simulink library "RobotG18_Blocos"  (R2016a)
settings: Solver=VariableStepAuto  StartTime=0.0  StopTime=10.0  RelTol=1e-3
settings Model: Creator=Catarina  LastModifiedBy=Catarina
settings GRTTargetCC: GeneratePreprocessorConditionals=Use local settings

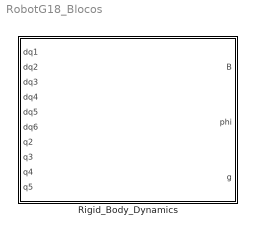
== system RobotG18_Blocos ==
  Rigid_Body_Dynamics : MATLAB Function  TreatAsAtomicUnit=on

== matlab function RobotG18_Blocos/Rigid_Body_Dynamics ==
  data: dq1 input; B output; dq2 input; dq3 input; dq4 input; dq5 input; dq6 input; q2 input; q3 input; q4 input; q5 input; phi output; g output
function [B,phi,g] = Rigid_Body_Dynamics(dq1,dq2,dq3,dq4,dq5,dq6,q2,q3,q4,q5)
%#codegen

%    This function was generated by the Symbolic Math Toolbox version 7.0.
%    17-May-2021 21:26:31

t2 = q2.*2.0;
t3 = q3.*2.0;
t4 = q4.*2.0;
t5 = q5.*2.0;
t6 = q2+q3+q4;
t7 = cos(t6);
t8 = q2+q3+q5;
t9 = sin(t8);
t10 = q2+q3-q5;
t11 = sin(t10);
t12 = q2+q3+q4+q5;
t13 = cos(t12);
t14 = t13.*2.24434e-4;
t15 = q2+q3;
t16 = sin(t15);
t17 = q2+q3+q4-q5;
t18 = cos(t17);
t19 = q2+q3+q4-t5;
t20 = cos(t19);
t21 = q2+q3+q4+t5;
t22 = cos(t21);
t23 = t22.*1.004271e-3;
t24 = q2-q5;
t25 = sin(t24);
t26 = q2+q5;
t27 = sin(t26);
t28 = t9.*6.284152e-3;
t29 = t27.*6.813175e-3;
t30 = sin(q2);
t31 = q4-q5;
t32 = sin(t31);
t33 = q3+q4+q5;
t34 = sin(t33);
t35 = cos(t5);
t36 = q3+q4-q5;
t37 = sin(t36);
t38 = q3+q4;
t39 = sin(t38);
t40 = q4+q5;
t41 = sin(t40);
t42 = cos(q3);
t43 = sin(q4);
t44 = t34.*6.813175e-3;
t45 = t41.*1.2568304e-2;
t46 = t42.*5.92297e-1;
t47 = t41.*6.284152e-3;
t48 = cos(q5);
t49 = t37.*6.813175e-3;
t50 = t32.*6.284152e-3;
t51 = t48.*2.75e-4;
t52 = t7.*(-8.11832e-3)+t14-t18.*3.270324e-3-t20.*1.004271e-3+t23;
t54 = t35.*2.008542e-3;
t53 = t43.*(-2.919616e-2)+t47-t50-t54+1.0090142e-2;
t55 = t7.*4.561084e-3;
t56 = t13.*3.270324e-3;
t57 = t18.*2.24434e-4;
t58 = t11.*(-6.284152e-3)-t25.*6.813175e-3+t28+t29+t55+t56+t57;
t60 = t48.*3.04589e-3;
t59 = t44+t47+t49+t50-t60;
t61 = dq2.^2;
t62 = sin(t17);
t63 = dq3.^2;
t64 = sin(t19);
t65 = sin(t21);
t66 = dq4.^2;
t67 = dq5.^2;
t68 = cos(t24);
t69 = cos(t8);
t70 = sin(t6);
t71 = cos(t10);
t72 = sin(t12);
t73 = cos(t15);
t74 = cos(t26);
t75 = sin(q5);
t76 = q3+q4+q5+t2;
t77 = cos(t76);
t78 = cos(t31);
t79 = q3+t2;
t80 = sin(t79);
t81 = -q5+t2+t3+t4;
t82 = t2+t3+t4+t5;
t83 = sin(t81);
t84 = t2+t3+t4-t5;
t85 = sin(t84);
t86 = sin(t82);
t87 = cos(t33);
t88 = t2+t3+t4;
t89 = sin(t88);
t90 = q3+q4-q5+t2;
t91 = q4+q5+t2+t3;
t92 = cos(t90);
t93 = cos(t91);
t94 = t2+t3;
t95 = sin(t94);
t96 = q3+q4+t2;
t97 = cos(t96);
t98 = cos(t36);
t99 = cos(t38);
t100 = cos(t40);
t101 = q4-q5+t2+t3;
t102 = cos(t101);
t103 = q5+t2+t3+t4;
t104 = sin(t103);
t105 = q4+t2+t3;
B = reshape([t32.*(-6.284152e-3)+t35.*1.004271e-3-t37.*6.813175e-3-t39.*3.1654e-2-t43.*2.919616e-2+t44+t46+t47+t48.*6.989516e-3+cos(t2).*1.2343024296875+cos(t79).*5.92297e-1-cos(t81).*1.522945e-3-cos(t82).*5.021355e-4-cos(t88).*2.630029e-3+cos(t94).*4.3975568975e-1+cos(t103).*1.522945e-3+sin(t76).*6.813175e-3-sin(t90).*6.813175e-3+sin(t91).*6.284152e-3-sin(t96).*3.1654e-2-sin(t101).*6.284152e-3-sin(t105).*2.919616e-2-cos(q5.*-2.0+t2+t3+t4).*5.021355e-4+1.8244887907375,t7.*(-8.11832e-3)-t11.*6.284152e-3+t14-t16.*6.2876312e-2-t18.*3.270324e-3-t20.*1.004271e-3+t23-t25.*6.813175e-3-t28-t29-t30.*2.9199618625e-1,t7.*(-8.11832e-3)-t11.*6.284152e-3+t14-t16.*6.2876312e-2-t18.*3.270324e-3-t20.*1.004271e-3+t23-t28,t52,t58,t70.*t75.*2.75e-4,t7.*(-8.11832e-3)-t9.*6.284152e-3-t11.*6.284152e-3+t14-t16.*6.2876312e-2-t18.*3.270324e-3-t20.*1.004271e-3+t23-t25.*6.813175e-3-t27.*6.813175e-3-t30.*2.9199618625e-1,t32.*(-1.2568304e-2)+t34.*1.362635e-2-t35.*2.008542e-3-t37.*1.362635e-2-t39.*6.3308e-2+t42.*1.184594-t43.*5.839232e-2+t45+3.377115380875,t32.*(-1.2568304e-2)-t35.*2.008542e-3-t39.*3.1654e-2-t43.*5.839232e-2+t44+t45+t46-t49+8.953005215e-1,t35.*(-2.008542e-3)-t39.*3.1654e-2-t43.*2.919616e-2+t44+t47-t49-t50+1.0090142e-2,t59,t51,t7.*(-8.11832e-3)-t9.*6.284152e-3-t11.*6.284152e-3+t14-t16.*6.2876312e-2-t18.*3.270324e-3-t20.*1.004271e-3+t23,t32.*(-1.2568304e-2)-t35.*2.008542e-3-t37.*6.813175e-3-t39.*3.1654e-2-t43.*5.839232e-2+t44+t45+t46+8.953005215e-1,t32.*(-1.2568304e-2)-t35.*2.008542e-3-t43.*5.839232e-2+t45+8.953005215e-1,t53,t47+t50-t60,t51,t52,t32.*(-6.284152e-3)-t35.*2.008542e-3-t37.*6.813175e-3-t39.*3.1654e-2-t43.*2.919616e-2+t44+t47+1.0090142e-2,t53,-t54+1.0090142e-2,-t60,t51,t58,t59,t47-t48.*3.04589e-3+t50,t48.*(-3.04589e-3),4.561084e-3,0.0,t13.*(-1.375e-4)+t18.*1.375e-4,t51,t51,t51,0.0,2.75e-4],[6,6]);
if nargout > 1
    t106 = cos(t105);
    t107 = sin(q3);
    t108 = dq1.^2;
    t109 = sin(t2);
    t110 = cos(q4);
    t111 = sin(t5);
    t112 = t67.*t75.*3.04589e-3;
    t113 = t95.*t108.*4.3975568975e-1;
    t114 = t66.*t100.*6.284152e-3;
    t115 = t67.*t100.*6.284152e-3;
    t116 = t102.*t108.*6.284152e-3;
    t117 = t104.*t108.*1.522945e-3;
    t118 = t106.*t108.*2.919616e-2;
    t119 = dq1.*dq6.*t62.*1.375e-4;
    t120 = dq2.*dq5.*t78.*1.2568304e-2;
    t121 = dq3.*dq5.*t78.*1.2568304e-2;
    t122 = dq4.*dq5.*t78.*1.2568304e-2;
    t123 = dq1.*dq5.*t70.*4.561084e-3;
    t124 = dq2.*dq5.*t111.*4.017084e-3;
    t125 = dq3.*dq5.*t111.*4.017084e-3;
    t126 = dq4.*dq5.*t111.*4.017084e-3;
    t127 = dq1.*dq5.*t71.*1.2568304e-2;
    t128 = dq1.*dq5.*t72.*3.04589e-3;
    t129 = dq2.*dq4.*t100.*1.2568304e-2;
    t130 = dq2.*dq5.*t100.*1.2568304e-2;
    t131 = dq3.*dq4.*t100.*1.2568304e-2;
    t132 = dq3.*dq5.*t100.*1.2568304e-2;
    t133 = dq4.*dq5.*t100.*1.2568304e-2;
    t134 = t92.*t108.*3.4065875e-3;
    t135 = t97.*t108.*1.5827e-2;
    t136 = t98.*t108.*3.4065875e-3;
    t137 = t61.*t98.*6.813175e-3;
    t138 = t99.*t108.*1.5827e-2;
    t139 = t61.*t99.*3.1654e-2;
    t140 = t78.*t108.*3.142076e-3;
    t141 = t61.*t78.*6.284152e-3;
    t142 = t63.*t78.*6.284152e-3;
    t143 = t102.*t108.*3.142076e-3;
    t144 = dq2.*dq3.*t78.*1.2568304e-2;
    t145 = cos(q2);
    phi = [t61.*t62.*3.270324e-3+t61.*t64.*1.004271e-3+t62.*t63.*3.270324e-3-t61.*t65.*1.004271e-3+t63.*t64.*1.004271e-3+t62.*t66.*3.270324e-3-t63.*t65.*1.004271e-3-t61.*t68.*6.813175e-3+t62.*t67.*2.24434e-4-t61.*t69.*6.284152e-3+t64.*t66.*1.004271e-3+t61.*t70.*8.11832e-3-t65.*t66.*1.004271e-3-t61.*t71.*6.284152e-3-t63.*t69.*6.284152e-3-t61.*t72.*2.24434e-4+t63.*t70.*8.11832e-3-t61.*t73.*6.2876312e-2-t63.*t71.*6.284152e-3-t61.*t74.*6.813175e-3-t63.*t72.*2.24434e-4+t67.*t68.*6.813175e-3-t63.*t73.*6.2876312e-2+t66.*t70.*8.11832e-3+t67.*t69.*6.284152e-3-t66.*t72.*2.24434e-4+t67.*t71.*6.284152e-3-t67.*t72.*3.270324e-3+t67.*t74.*6.813175e-3-t61.*t145.*2.9199618625e-1+dq2.*dq3.*t62.*6.540648e-3+dq2.*dq4.*t62.*6.540648e-3+dq2.*dq3.*t64.*2.008542e-3-dq2.*dq5.*t62.*3.494758e-3+dq3.*dq4.*t62.*6.540648e-3-dq2.*dq3.*t65.*2.008542e-3+dq2.*dq4.*t64.*2.008542e-3-dq2.*dq6.*t62.*1.375e-4-dq3.*dq5.*t62.*3.494758e-3-dq2.*dq4.*t65.*2.008542e-3-dq2.*dq5.*t64.*2.008542e-3+dq3.*dq4.*t64.*2.008542e-3-dq3.*dq6.*t62.*1.375e-4-dq4.*dq5.*t62.*3.494758e-3-dq2.*dq5.*t65.*2.008542e-3-dq3.*dq4.*t65.*2.008542e-3-dq3.*dq5.*t64.*2.008542e-3-dq4.*dq6.*t62.*1.375e-4-dq3.*dq5.*t65.*2.008542e-3-dq4.*dq5.*t64.*2.008542e-3+dq5.*dq6.*t62.*1.375e-4-dq2.*dq3.*t69.*1.2568304e-2-dq4.*dq5.*t65.*2.008542e-3+dq2.*dq3.*t70.*1.623664e-2-dq2.*dq3.*t71.*1.2568304e-2+dq2.*dq4.*t70.*1.623664e-2-dq2.*dq3.*t72.*4.48868e-4-dq2.*dq5.*t70.*4.561084e-3+dq3.*dq4.*t70.*1.623664e-2-dq2.*dq3.*t73.*1.25752624e-1-dq2.*dq4.*t72.*4.48868e-4-dq3.*dq5.*t70.*4.561084e-3-dq2.*dq5.*t72.*3.494758e-3-dq3.*dq4.*t72.*4.48868e-4-dq4.*dq5.*t70.*4.561084e-3+dq1.*dq2.*t77.*1.362635e-2+dq2.*dq6.*t72.*1.375e-4-dq3.*dq5.*t72.*3.494758e-3+dq1.*dq3.*t77.*6.813175e-3-dq1.*dq5.*t75.*6.989516e-3+dq3.*dq6.*t72.*1.375e-4-dq4.*dq5.*t72.*3.494758e-3+dq1.*dq4.*t77.*6.813175e-3+dq4.*dq6.*t72.*1.375e-4-dq1.*dq2.*t80.*1.184594-dq1.*dq4.*t78.*6.284152e-3+dq1.*dq5.*t77.*6.813175e-3+dq5.*dq6.*t72.*1.375e-4-dq1.*dq3.*t80.*5.92297e-1+dq1.*dq5.*t78.*6.284152e-3+dq1.*dq2.*t83.*3.04589e-3+dq1.*dq3.*t83.*3.04589e-3+dq1.*dq2.*t85.*1.004271e-3+dq1.*dq4.*t83.*3.04589e-3+dq1.*dq2.*t86.*1.004271e-3+dq1.*dq3.*t85.*1.004271e-3-dq1.*dq5.*t83.*1.522945e-3+dq1.*dq3.*t86.*1.004271e-3+dq1.*dq4.*t85.*1.004271e-3+dq1.*dq3.*t87.*6.813175e-3+dq1.*dq4.*t86.*1.004271e-3-dq1.*dq5.*t85.*1.004271e-3+dq1.*dq2.*t89.*5.260058e-3+dq1.*dq4.*t87.*6.813175e-3+dq1.*dq5.*t86.*1.004271e-3+dq1.*dq3.*t89.*5.260058e-3+dq1.*dq5.*t87.*6.813175e-3+dq1.*dq4.*t89.*5.260058e-3-dq1.*dq2.*t92.*1.362635e-2+dq1.*dq2.*t93.*1.2568304e-2-dq1.*dq3.*t92.*6.813175e-3+dq1.*dq3.*t93.*1.2568304e-2-dq1.*dq4.*t92.*6.813175e-3-dq1.*dq2.*t95.*8.795113794999999e-1+dq1.*dq4.*t93.*6.284152e-3+dq1.*dq5.*t92.*6.813175e-3-dq1.*dq3.*t95.*8.795113794999999e-1+dq1.*dq5.*t93.*6.284152e-3-dq1.*dq2.*t97.*6.3308e-2-dq1.*dq3.*t97.*3.1654e-2-dq1.*dq3.*t98.*6.813175e-3-dq1.*dq4.*t97.*3.1654e-2-dq1.*dq3.*t99.*3.1654e-2-dq1.*dq4.*t98.*6.813175e-3-dq1.*dq4.*t99.*3.1654e-2+dq1.*dq5.*t98.*6.813175e-3-dq1.*dq2.*t102.*1.2568304e-2+dq1.*dq4.*t100.*6.284152e-3-dq1.*dq3.*t102.*1.2568304e-2+dq1.*dq5.*t100.*6.284152e-3-dq1.*dq2.*t104.*3.04589e-3-dq1.*dq4.*t102.*6.284152e-3-dq1.*dq3.*t104.*3.04589e-3+dq1.*dq5.*t102.*6.284152e-3-dq1.*dq2.*t106.*5.839232e-2-dq1.*dq4.*t104.*3.04589e-3-dq1.*dq3.*t106.*5.839232e-2-dq1.*dq5.*t104.*1.522945e-3-dq1.*dq3.*t107.*5.92297e-1-dq1.*dq4.*t106.*2.919616e-2-dq1.*dq2.*t109.*2.468604859375-dq1.*dq4.*t110.*2.919616e-2-dq1.*dq5.*t111.*2.008542e-3;t112+t113+t114+t115+t116+t117+t118+t119+t120+t121+t122+t123+t124+t125+t126+t127+t128+t129+t130+t131+t132+t133-t66.*t78.*6.284152e-3-t67.*t78.*6.284152e-3+t63.*t87.*6.813175e-3+t66.*t87.*6.813175e-3+t67.*t87.*6.813175e-3-t63.*t98.*6.813175e-3-t63.*t99.*3.1654e-2-t66.*t98.*6.813175e-3-t66.*t99.*3.1654e-2-t67.*t98.*6.813175e-3-t63.*t107.*5.92297e-1-t66.*t110.*2.919616e-2-t77.*t108.*6.813175e-3+t80.*t108.*5.92297e-1-t83.*t108.*1.522945e-3-t85.*t108.*5.021355e-4-t86.*t108.*5.021355e-4-t89.*t108.*2.630029e-3+t92.*t108.*6.813175e-3-t93.*t108.*6.284152e-3+t97.*t108.*3.1654e-2+t108.*t109.*1.2343024296875-dq1.*dq5.*t62.*3.04589e-3-dq1.*dq5.*t64.*2.008542e-3-dq1.*dq5.*t65.*2.008542e-3+dq1.*dq5.*t68.*1.362635e-2-dq1.*dq5.*t69.*1.2568304e-2-dq1.*dq6.*t72.*1.375e-4-dq1.*dq5.*t74.*1.362635e-2-dq2.*dq4.*t78.*1.2568304e-2-dq3.*dq4.*t78.*1.2568304e-2-dq5.*dq6.*t75.*2.75e-4+dq2.*dq3.*t87.*1.362635e-2+dq2.*dq4.*t87.*1.362635e-2+dq2.*dq5.*t87.*1.362635e-2+dq3.*dq4.*t87.*1.362635e-2+dq3.*dq5.*t87.*1.362635e-2+dq4.*dq5.*t87.*1.362635e-2-dq2.*dq3.*t98.*1.362635e-2-dq2.*dq3.*t99.*6.3308e-2-dq2.*dq4.*t98.*1.362635e-2-dq2.*dq4.*t99.*6.3308e-2+dq2.*dq5.*t98.*1.362635e-2-dq3.*dq4.*t98.*1.362635e-2-dq3.*dq4.*t99.*6.3308e-2+dq3.*dq5.*t98.*1.362635e-2+dq4.*dq5.*t98.*1.362635e-2-dq2.*dq3.*t107.*1.184594-dq2.*dq4.*t110.*5.839232e-2-dq3.*dq4.*t110.*5.839232e-2;t112+t113+t114+t115+t116+t117+t118+t119+t120+t121+t122+t123+t124+t125+t126+t127+t128+t129+t130+t131+t132+t133+t134+t135+t136+t137+t138+t139-t66.*t78.*6.284152e-3-t67.*t78.*6.284152e-3-t61.*t87.*6.813175e-3+t61.*t107.*5.92297e-1-t66.*t110.*2.919616e-2-t77.*t108.*3.4065875e-3+t80.*t108.*2.961485e-1-t83.*t108.*1.522945e-3-t85.*t108.*5.021355e-4-t86.*t108.*5.021355e-4-t87.*t108.*3.4065875e-3-t89.*t108.*2.630029e-3-t93.*t108.*6.284152e-3+t107.*t108.*2.961485e-1-dq1.*dq5.*t62.*3.04589e-3-dq1.*dq5.*t64.*2.008542e-3-dq1.*dq5.*t65.*2.008542e-3-dq1.*dq5.*t69.*1.2568304e-2-dq1.*dq6.*t72.*1.375e-4-dq2.*dq4.*t78.*1.2568304e-2-dq3.*dq4.*t78.*1.2568304e-2-dq5.*dq6.*t75.*2.75e-4-dq2.*dq4.*t110.*5.839232e-2-dq3.*dq4.*t110.*5.839232e-2;t112+t117+t119+t123+t124+t125+t126+t128+t134+t135+t136+t137+t138+t139+t140+t141+t142+t143+t144-t61.*t87.*6.813175e-3-t61.*t100.*6.284152e-3-t63.*t100.*6.284152e-3+t61.*t110.*2.919616e-2+t63.*t110.*2.919616e-2-t77.*t108.*3.4065875e-3-t83.*t108.*1.522945e-3-t85.*t108.*5.021355e-4-t86.*t108.*5.021355e-4-t87.*t108.*3.4065875e-3-t89.*t108.*2.630029e-3-t93.*t108.*3.142076e-3-t100.*t108.*3.142076e-3+t106.*t108.*1.459808e-2+t108.*t110.*1.459808e-2-dq1.*dq5.*t62.*3.04589e-3-dq1.*dq5.*t64.*2.008542e-3-dq1.*dq5.*t65.*2.008542e-3-dq1.*dq6.*t72.*1.375e-4-dq5.*dq6.*t75.*2.75e-4-dq2.*dq3.*t100.*1.2568304e-2+dq2.*dq3.*t110.*5.839232e-2;-t119-t134-t136-t137-t140-t141-t142-t143-t144-t61.*t87.*6.813175e-3-t61.*t100.*6.284152e-3-t63.*t100.*6.284152e-3-t61.*t111.*2.008542e-3-t63.*t111.*2.008542e-3-t66.*t111.*2.008542e-3+t75.*t108.*3.494758e-3-t77.*t108.*3.4065875e-3+t83.*t108.*7.614725e-4+t85.*t108.*5.021355e-4-t86.*t108.*5.021355e-4-t87.*t108.*3.4065875e-3-t93.*t108.*3.142076e-3-t100.*t108.*3.142076e-3+t104.*t108.*7.614725e-4+t108.*t111.*1.004271e-3+dq1.*dq2.*t62.*3.04589e-3+dq1.*dq3.*t62.*3.04589e-3+dq1.*dq2.*t64.*2.008542e-3+dq1.*dq4.*t62.*3.04589e-3+dq1.*dq2.*t65.*2.008542e-3+dq1.*dq3.*t64.*2.008542e-3+dq1.*dq3.*t65.*2.008542e-3+dq1.*dq4.*t64.*2.008542e-3+dq1.*dq4.*t65.*2.008542e-3-dq1.*dq2.*t68.*1.362635e-2+dq1.*dq2.*t69.*1.2568304e-2-dq1.*dq2.*t70.*4.561084e-3+dq1.*dq3.*t69.*1.2568304e-2-dq1.*dq2.*t71.*1.2568304e-2-dq1.*dq3.*t70.*4.561084e-3-dq1.*dq2.*t72.*3.04589e-3-dq1.*dq3.*t71.*1.2568304e-2-dq1.*dq4.*t70.*4.561084e-3-dq1.*dq3.*t72.*3.04589e-3+dq1.*dq2.*t74.*1.362635e-2-dq1.*dq4.*t72.*3.04589e-3-dq1.*dq6.*t72.*1.375e-4+dq2.*dq6.*t75.*2.75e-4+dq3.*dq6.*t75.*2.75e-4+dq4.*dq6.*t75.*2.75e-4-dq2.*dq3.*t100.*1.2568304e-2-dq2.*dq3.*t111.*4.017084e-3-dq2.*dq4.*t111.*4.017084e-3-dq3.*dq4.*t111.*4.017084e-3;dq2.*dq5.*t75.*(-2.75e-4)-dq3.*dq5.*t75.*2.75e-4-dq4.*dq5.*t75.*2.75e-4+dq1.*dq2.*t7.*t75.*2.75e-4+dq1.*dq3.*t7.*t75.*2.75e-4+dq1.*dq4.*t7.*t75.*2.75e-4+dq1.*dq5.*t48.*t70.*2.75e-4];
end
if nargout > 2
    t146 = t72.*1.5726411e-1;
    t147 = t73.*1.36716084e1;
    g = [0.0;t62.*(-1.5726411e-1)-t70.*7.306488e-1+t145.*4.67942027625e1+t146+t147;t62.*(-1.5726411e-1)-t70.*7.306488e-1+t146+t147;t70.*(-7.306488e-1)+t7.*t75.*3.1452822e-1;t48.*t70.*3.1452822e-1;0.0];
end
